simulink model "ejemplo3Z_N"  (R2019a)
settings: Solver=VariableStepAuto  StartTime=0.0  StopTime=10.0  RelTol=1e-3
settings Model: Creator=juanjosegdoj  LastModifiedBy=juanjosegdoj

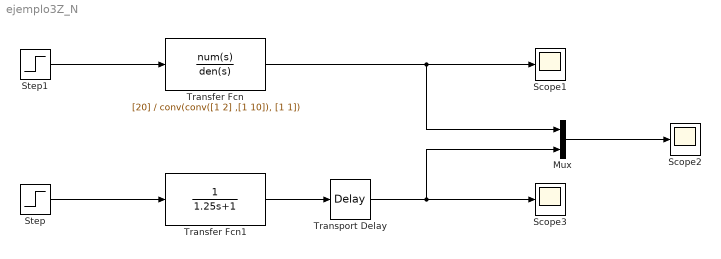
== system ejemplo3Z_N ==
  Mux : Mux  Inputs=2
  Scope1 : Scope
  Scope2 : Scope
  Scope3 : Scope
  Step : Step  Time=0  SampleTime=0
  Step1 : Step  Time=0  SampleTime=0
  Transfer Fcn : TransferFcn  Numerator=[20]  Denominator=conv(conv([1 2] ,[1 10]), [1 1])
  Transfer Fcn1 : TransferFcn  Denominator=[1.25 1]
  Transport Delay : TransportDelay
  wires:
  Step1/1 -> Transfer Fcn/1
  Transfer Fcn/1 -> Mux/1, Scope1/1
  Mux/1 -> Scope2/1
  Step/1 -> Transfer Fcn1/1
  Transfer Fcn1/1 -> Transport Delay/1
  Transport Delay/1 -> Scope3/1, Mux/2
